simulink model "Vereinzelung"  (R2020b)
settings: Solver=VariableStepAuto  StartTime=0.0  StopTime=10.0  RelTol=1e-3
settings Model: Creator=kaebi  LastModifiedBy=kaebi
settings ConfigComp: PLC_TargetIDE=twincat3

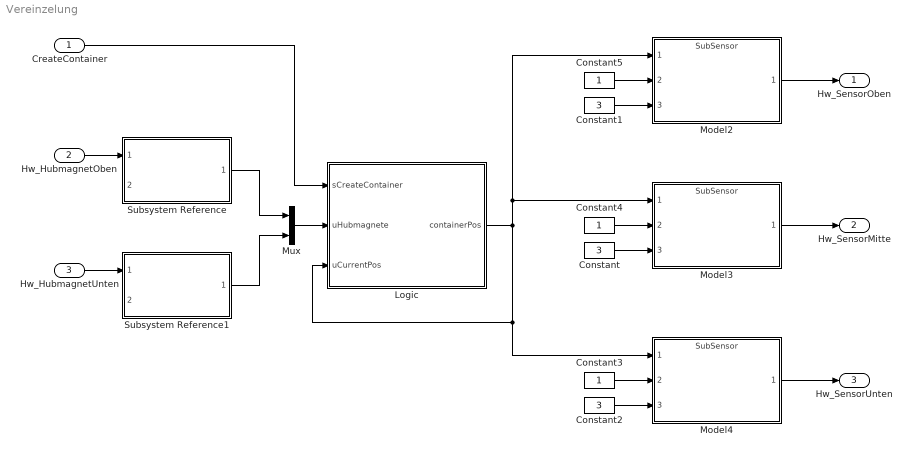
== system Vereinzelung ==
  CreateContainer : Inport
  Hw_HubmagnetOben : Inport  Port=2
  Hw_HubmagnetUnten : Inport  Port=3
  Constant : Constant  Value=3
  Constant1 : Constant  Value=3
  Constant2 : Constant  Value=3
  Constant3 : Constant
  Constant4 : Constant
  Constant5 : Constant
  Logic : MATLAB Function  TreatAsAtomicUnit=on
  Model2 : ModelReference  ModelNameDialog=SubSensor.slx  SimulationMode=Normal  ModelReferenceVersion=1.1
  Model3 : ModelReference  ModelNameDialog=SubSensor.slx  SimulationMode=Normal  ModelReferenceVersion=1.1
  Model4 : ModelReference  ModelNameDialog=SubSensor.slx  SimulationMode=Normal  ModelReferenceVersion=1.1
  Mux : Mux  Inputs=2
  Subsystem Reference : Subsystem  ReferencedSubsystem=SubSystemHubmagnet
  Subsystem Reference1 : Subsystem  ReferencedSubsystem=SubSystemHubmagnet
  Hw_SensorOben : Outport
  Hw_SensorMitte : Outport  Port=2
  Hw_SensorUnten : Outport  Port=3
  wires:
  Subsystem Reference1/1 -> Mux/2
  Constant/1 -> Model3/3
  Constant5/1 -> Model2/2
  Constant2/1 -> Model4/3
  Constant3/1 -> Model4/2
  Model3/1 -> Hw_SensorMitte/1
  Mux/1 -> Logic/2(uHubmagnete)
  Constant1/1 -> Model2/3
  Subsystem Reference/1 -> Mux/1
  Hw_HubmagnetUnten/1 -> Subsystem Reference1/1
  Hw_HubmagnetOben/1 -> Subsystem Reference/1
  Model4/1 -> Hw_SensorUnten/1
  Constant4/1 -> Model3/2
  Logic/1(containerPos) -> Model3/1, Model2/1, Model4/1, Logic/3(uCurrentPos)
  CreateContainer/1 -> Logic/1(sCreateContainer)
  Model2/1 -> Hw_SensorOben/1

== matlab function Vereinzelung/Logic ==
  data: sCreateContainer input; uHubmagnete input; containerPos output; uCurrentPos input
function containerPos = LogikVereinzelung(sCreateContainer, uHubmagnete, uCurrentPos)

    

    containerPos = uCurrentPos +1;    
end
